simulink library "ADCS_lib"  (R2019a)
settings: Solver=VariableStepAuto  StartTime=0.0  StopTime=10.0  RelTol=1e-3
undefined symbols (not defined in the file): D_distri, G_g, G_s, G_t, Gs, I_rw, I_vscmg, I_w, J_w, K, Kc, Ki, Kp, Kv, m, OMEGA_0, P, quat_0, smiData, X, Y, Z
libraries: sm_lib x31, aerolibutil x15, nesl_utility x13, sharedtransform x4, $bdroot x2
(part 1 of 3)
settings Model: Creator=steven  LastModifiedBy=zhang
settings DataIOCC: ReturnWorkspaceOutputs=off
settings DebuggingCC: ArithmeticOperatorsInVariantConditions=warning
settings SFSimCC: SimUseLocalCustomCode=off
settings RTWCC: RTWUseLocalCustomCode=off

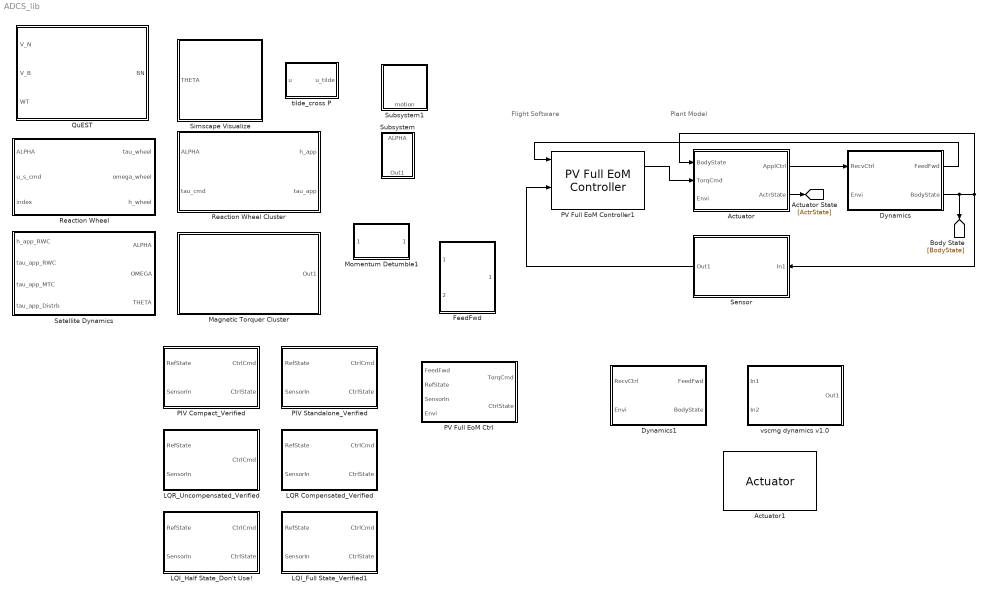
== system ADCS_lib ==
  note: Flight Software
  note: Plant Model
  Actuator : Subsystem
  Actuator1 : $bdroot/Actuator  SystemSampleTime=-1
  Dynamics : Subsystem
  Dynamics1 : Subsystem  AncestorBlock=ADCS_lib/Dynamics
  FeedFwd : Subsystem
  LQI_Full State_Verified1 : Subsystem  AncestorBlock=ADCS_lib/Full EoM Controller
      mask help:
      | Gains
      |
      | 1U
      | Kc = [eye(3).*[2.5;2.5;2.5]  eye(3).*[5;5;5]];
      | Ki  = [eye(3).*[1.2 1.2 1.2]  eye(3).*[3;3;3]];
      | Set large Ki velocity gain to surpress oscillation, x & z axis gains have the most effect
      |
      | 3U
  LQI_Half State_Don't Use! : Subsystem  AncestorBlock=ADCS_lib/Full EoM Controller
  LQR Compensated_Verified : Subsystem  AncestorBlock=ADCS_lib/PIV
  LQR_Uncompensated_Verified : Subsystem  AncestorBlock=ADCS_lib/LQR
  Magnetic Torquer Cluster : Subsystem
      mask Display: image('magnetic torquer cluster.png');
  Momentum Detumble1 : Subsystem
  PIV Compact_Verified : Subsystem  AncestorBlock=ADCS_lib/Full EoM Controller
  PIV Standalone_Verified : Subsystem  AncestorBlock=ADCS_lib/Full EoM Controller
  PV Full EoM Controller1 : $bdroot/PV Full EoM Controller  SystemSampleTime=-1  SSRTWFcnClass=[]
  PV Full EoM Ctrl : Subsystem  AncestorBlock=ADCS_lib/Full EoM Controller
  QuEST : MATLAB Function  TreatAsAtomicUnit=on  mask(QUEST Attitude Estimation){}
      mask help:
      | Estimate spacecraft attitude using QUEST algorithm
      |
      | Input: sensor measurement in inertia frame V_N
      | V_N = [x1 x2 x3 x4 x5 ... ;
      |              y1 y2 y3 y4 y5 ... ;
      |              z1 z2  z3 z4 z5 ...  ]
      |
      |             sensor measurement in body frame V_B
      | V_B = [x1 x2 x3 x4 x5 ... ;
      |             y1 y2 y3 y4 y5 ... ;
      |             z1 z2  z3 z4 z5 ...  ]
      |
      |             sensor weight wt
      | wt = [wt1 wt2 wt3 wt4 wt5 ...]
      |
      | Output: attitude [BN] in quaternion
      mask init:
      | clear all;
      | clc;
  Reaction Wheel : MATLAB Function  TreatAsAtomicUnit=on  mask(Single Reaction Wheel){}
      mask help:
      | INPUT
      | ALPHA ==> spacecraft angular acceleration (vector)
      | u_s ==> motor torque command magnitude for individual wheel in g_s direction (scalar)
      | index ==> select which wheel (1-4) (scalar)
      |
      | OUTPUT
      | tau_wheel ==> individual applied torque magnitude to spacecraft body in g_s direction (scalar)
      | omega_wheel ==> individual wheel angular velocity magnitude in g_s direction (scalar)
  Reaction Wheel Cluster : Subsystem  mask(Reaction Wheel Cluster){}
      mask Display: image('reaction wheel cluster.png');
  Satellite Dynamics : Subsystem
      mask Display: image('3u cubesat.png');
  Sensor : Subsystem
  Simscape Visualize : Subsystem
      mask Display: image('camera.png');
  Subsystem : Subsystem
  Subsystem1 : Subsystem
      mask Display: image('camera.png');
  tilde_cross P : MATLAB Function  TreatAsAtomicUnit=on
  vscmg dynamics v1.0 : Subsystem
  wires:
  ? -> PV Full EoM Controller1/2
  ? -> PV Full EoM Controller1/4, Actuator/3(Envi), Dynamics/2(Envi)
  PV Full EoM Controller1/1 -> Actuator/2(TorqCmd)
  Sensor/1(Out1) -> PV Full EoM Controller1/3
  Actuator/1(ApplCtrl) -> Dynamics/1(RecvCtrl)
  Dynamics/1(FeedFwd) -> PV Full EoM Controller1/1
  Dynamics/2(BodyState) -> Sensor/1(In1), Actuator/1(BodyState), [BodyState]
  Actuator/2(ActrState) -> [ActrState]

== system ADCS_lib/Actuator ==
  In Bus Element3 : Inport  PortName=BodyState  Element=b_a_b/n
  In Bus Element2 : Inport  PortName=BodyState  Element=b_w_b/n
  In Bus Element : Inport  Port=2  PortName=TorqCmd  Element=b_t_cmd_rwc
  In Bus Element1 : Inport  Port=2  PortName=TorqCmd  Element=b_t_cmd_mtc
  In Bus Element4 : Inport  Port=3  PortName=Envi  Element=b_t_dstb
  Magnetic Torquer Cluster : Subsystem
  Reaction Wheel Cluster : Subsystem
  Out Bus Element : Outport  PortName=ApplCtrl  Element=h_s
  Out Bus Element1 : Outport  PortName=ApplCtrl  Element=u_s
  Out Bus Element2 : Outport  PortName=ApplCtrl  Element=mtc
  Out Bus Element3 : Outport  Port=2  PortName=ActrState  Element=w_rw
  Out Bus Element4 : Outport  Port=2  PortName=ActrState  Element=t_mtc
  wires:
  In Bus Element/1 -> Reaction Wheel Cluster/3(b_t_cmd_rwc)
  In Bus Element1/1 -> Out Bus Element4/1, Magnetic Torquer Cluster/1(b_t_cmd_mtc)
  In Bus Element2/1 -> Reaction Wheel Cluster/1(b_w_b/n)
  In Bus Element3/1 -> Reaction Wheel Cluster/2(b_a_b/n)
  Reaction Wheel Cluster/1(h_s) -> Out Bus Element/1
  Reaction Wheel Cluster/2(u_s) -> Out Bus Element1/1
  Magnetic Torquer Cluster/1(Out1) -> Out Bus Element2/1
  In Bus Element4/1 -> Magnetic Torquer Cluster/2(Envi)
  Reaction Wheel Cluster/3(omega_w) -> Out Bus Element3/1

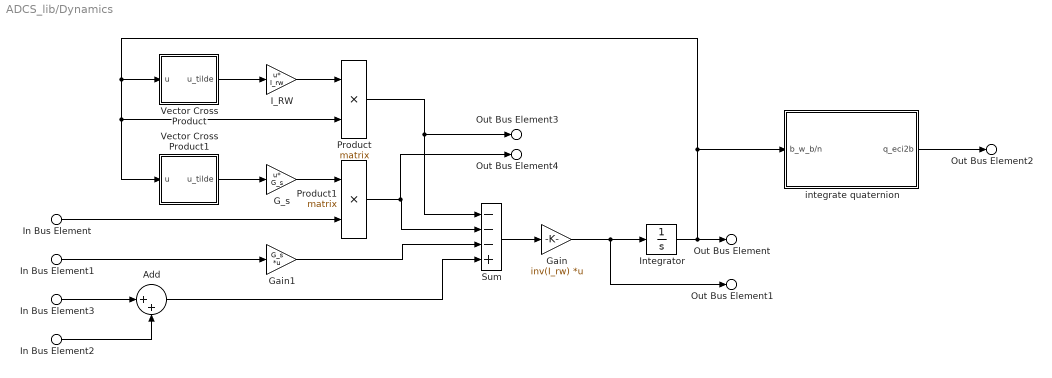
== system ADCS_lib/Dynamics ==
  In Bus Element1 : Inport  PortName=RecvCtrl  Element=u_s
  In Bus Element : Inport  PortName=RecvCtrl  Element=h_s
  In Bus Element3 : Inport  PortName=RecvCtrl  Element=mtc
  In Bus Element2 : Inport  Port=2  PortName=Envi  Element=b_t_dstb
  Add : Sum  Inputs=|++
  G_s : Gain  Gain=G_s  Multiplication=Matrix(u*K)
  Gain : Gain  Gain=inv(I_rw)  Multiplication=Matrix(K*u)
  Gain1 : Gain  Gain=G_s  Multiplication=Matrix(K*u)
  I_RW : Gain  Gain=I_rw  Multiplication=Matrix(u*K)
  Integrator : Integrator  InitialCondition=OMEGA_0
  Product : Product  Multiplication=Matrix(*)
  Product1 : Product  Multiplication=Matrix(*)
  Sum : Sum  Inputs=---+
  Vector Cross Product : MATLAB Function  TreatAsAtomicUnit=on
  Vector Cross Product1 : MATLAB Function  TreatAsAtomicUnit=on
  integrate quaternion : Subsystem
  Out Bus Element3 : Outport  PortName=FeedFwd  Element=1
  Out Bus Element4 : Outport  PortName=FeedFwd  Element=2
  Out Bus Element : Outport  Port=2  PortName=BodyState  Element=b_w_b/n
  Out Bus Element1 : Outport  Port=2  PortName=BodyState  Element=b_a_b/n
  Out Bus Element2 : Outport  Port=2  PortName=BodyState  Element=q_eci2b
  wires:
  In Bus Element2/1 -> Add/2
  Add/1 -> Sum/4
  In Bus Element3/1 -> Add/1
  Gain1/1 -> Sum/3
  In Bus Element1/1 -> Gain1/1
  Product1/1 -> Out Bus Element4/1, Sum/2
  In Bus Element/1 -> Product1/2
  G_s/1 -> Product1/1
  Vector Cross Product1/1(u_tilde) -> G_s/1
  Product/1 -> Out Bus Element3/1, Sum/1
  I_RW/1 -> Product/1
  Vector Cross Product/1(u_tilde) -> I_RW/1
  Integrator/1 -> Out Bus Element/1, integrate quaternion/1(b_w_b/n), Product/2, Vector Cross Product1/1(u), Vector Cross Product/1(u)
  Gain/1 -> Out Bus Element1/1, Integrator/1
  Sum/1 -> Gain/1
  integrate quaternion/1(q_eci2b) -> Out Bus Element2/1

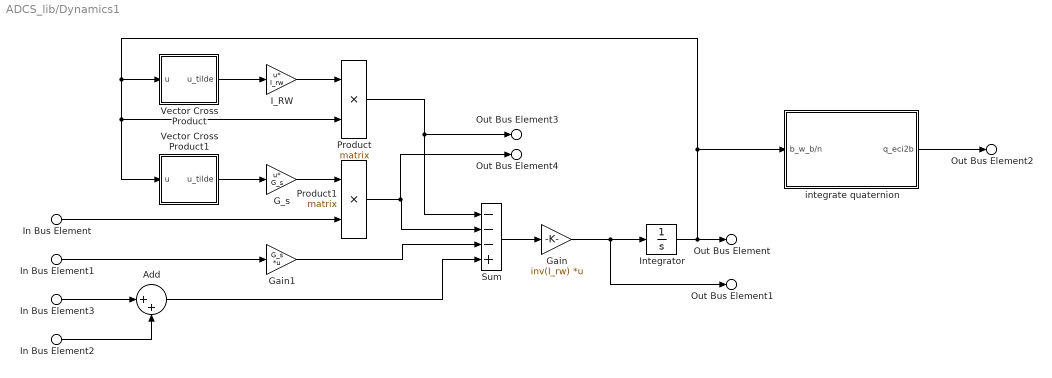
== system ADCS_lib/Dynamics1 ==
  In Bus Element1 : Inport  PortName=RecvCtrl  Element=u_s
  In Bus Element : Inport  PortName=RecvCtrl  Element=h_s
  In Bus Element3 : Inport  PortName=RecvCtrl  Element=mtc
  In Bus Element2 : Inport  Port=2  PortName=Envi  Element=b_t_dstb
  Add : Sum  Inputs=|++
  G_s : Gain  Gain=G_s  Multiplication=Matrix(u*K)
  Gain : Gain  Gain=inv(I_rw)  Multiplication=Matrix(K*u)
  Gain1 : Gain  Gain=G_s  Multiplication=Matrix(K*u)
  I_RW : Gain  Gain=I_rw  Multiplication=Matrix(u*K)
  Integrator : Integrator  InitialCondition=OMEGA_0
  Product : Product  Multiplication=Matrix(*)
  Product1 : Product  Multiplication=Matrix(*)
  Sum : Sum  Inputs=---+
  Vector Cross Product : MATLAB Function  TreatAsAtomicUnit=on
  Vector Cross Product1 : MATLAB Function  TreatAsAtomicUnit=on
  integrate quaternion : Subsystem
  Out Bus Element3 : Outport  PortName=FeedFwd  Element=1
  Out Bus Element4 : Outport  PortName=FeedFwd  Element=2
  Out Bus Element : Outport  Port=2  PortName=BodyState  Element=b_w_b/n
  Out Bus Element1 : Outport  Port=2  PortName=BodyState  Element=b_a_b/n
  Out Bus Element2 : Outport  Port=2  PortName=BodyState  Element=q_eci2b
  wires:
  integrate quaternion/1(q_eci2b) -> Out Bus Element2/1
  Sum/1 -> Gain/1
  Gain/1 -> Integrator/1, Out Bus Element1/1
  Integrator/1 -> Vector Cross Product/1(u), Vector Cross Product1/1(u), Product/2, integrate quaternion/1(b_w_b/n), Out Bus Element/1
  Vector Cross Product/1(u_tilde) -> I_RW/1
  I_RW/1 -> Product/1
  Product/1 -> Sum/1, Out Bus Element3/1
  Vector Cross Product1/1(u_tilde) -> G_s/1
  G_s/1 -> Product1/1
  In Bus Element/1 -> Product1/2
  Product1/1 -> Sum/2, Out Bus Element4/1
  In Bus Element1/1 -> Gain1/1
  Gain1/1 -> Sum/3
  In Bus Element3/1 -> Add/1
  Add/1 -> Sum/4
  In Bus Element2/1 -> Add/2

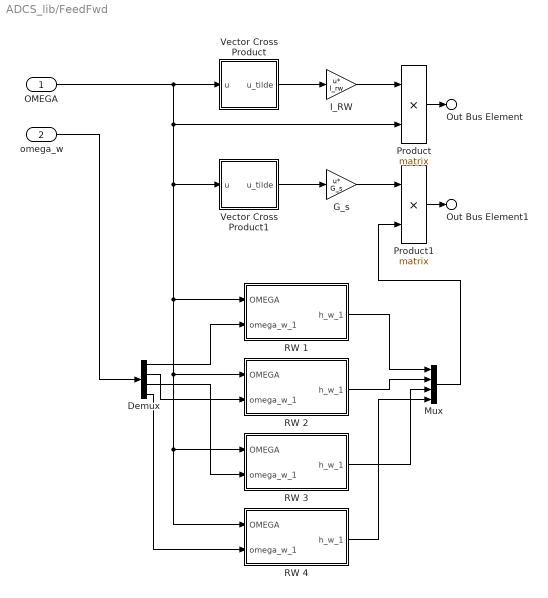
== system ADCS_lib/FeedFwd ==
  OMEGA : Inport
  omega_w : Inport  Port=2
  Demux : Demux
  G_s : Gain  Gain=G_s  Multiplication=Matrix(u*K)
  I_RW : Gain  Gain=I_rw  Multiplication=Matrix(u*K)
  Mux : Mux
  Product : Product  Multiplication=Matrix(*)
  Product1 : Product  Multiplication=Matrix(*)
  RW 1 : Subsystem
  RW 2 : Subsystem
  RW 3 : Subsystem
  RW 4 : Subsystem
  Vector Cross Product : MATLAB Function  TreatAsAtomicUnit=on
  Vector Cross Product1 : MATLAB Function  TreatAsAtomicUnit=on
  Out Bus Element : Outport  PortName=FeedFwd  Element=1
  Out Bus Element1 : Outport  PortName=FeedFwd  Element=2
  wires:
  Demux/2 -> RW 2/2(omega_w_1)
  RW 2/1(h_w_1) -> Mux/2
  Demux/4 -> RW 4/2(omega_w_1)
  OMEGA/1 -> Product/2, RW 4/1(OMEGA), RW 3/1(OMEGA), RW 2/1(OMEGA), RW 1/1(OMEGA), Vector Cross Product1/1(u), Vector Cross Product/1(u)
  Mux/1 -> Product1/2
  RW 4/1(h_w_1) -> Mux/4
  Demux/1 -> RW 1/2(omega_w_1)
  RW 1/1(h_w_1) -> Mux/1
  RW 3/1(h_w_1) -> Mux/3
  Demux/3 -> RW 3/2(omega_w_1)
  Vector Cross Product/1(u_tilde) -> I_RW/1
  Product/1 -> Out Bus Element/1
  I_RW/1 -> Product/1
  G_s/1 -> Product1/1
  Vector Cross Product1/1(u_tilde) -> G_s/1
  omega_w/1 -> Demux/1
  Product1/1 -> Out Bus Element1/1

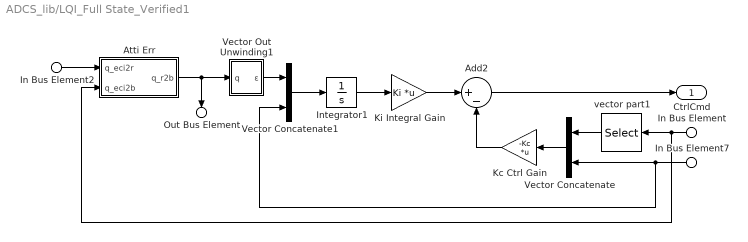
== system ADCS_lib/LQI_Full State_Verified1 ==
  In Bus Element2 : Inport  PortName=RefState  Element=q_eci2r
  In Bus Element : Inport  Port=2  PortName=SensorIn  Element=q_eci2b
  In Bus Element7 : Inport  Port=2  PortName=SensorIn  Element=b_w_b/n
  Add2 : Sum  Inputs=|+-
  Atti Err : Subsystem  AncestorBlock=ADCS_lib/PIV/Atti Err
  Integrator1 : Integrator
  Kc Ctrl Gain : Gain  Gain=-Kc  Multiplication=Matrix(K*u)
  Ki Integral Gain : Gain  Gain=Ki  Multiplication=Matrix(K*u)
  Vector Concatenate : Concatenate
  Vector Concatenate1 : Concatenate
  Vector Out Unwinding1 : Subsystem
  vector part1 : Selector  InputPortWidth=4  IndexOptions=Index vector (dialog)  Indices=[2 3 4]  OutputSizes=1
  CtrlCmd : Outport
  Out Bus Element : Outport  Port=2  PortName=CtrlState  Element=q_r2b
  wires:
  Vector Concatenate1/1 -> Integrator1/1
  Vector Out Unwinding1/1(ε) -> Vector Concatenate1/1
  In Bus Element7/1 -> Vector Concatenate1/2, Vector Concatenate/2
  Vector Concatenate/1 -> Kc Ctrl Gain/1
  vector part1/1 -> Vector Concatenate/1
  Integrator1/1 -> Ki Integral Gain/1
  Add2/1 -> CtrlCmd/1
  Kc Ctrl Gain/1 -> Add2/2
  In Bus Element2/1 -> Atti Err/1(q_eci2r)
  In Bus Element/1 -> Atti Err/2(q_eci2b), vector part1/1
  Atti Err/1(q_r2b) -> Vector Out Unwinding1/1(q), Out Bus Element/1
  Ki Integral Gain/1 -> Add2/1

== system ADCS_lib/LQI_Half State_Don't Use! ==
  In Bus Element2 : Inport  PortName=RefState  Element=q_eci2r
  In Bus Element : Inport  Port=2  PortName=SensorIn  Element=q_eci2b
  In Bus Element7 : Inport  Port=2  PortName=SensorIn  Element=b_w_b/n
  Add2 : Sum  Inputs=|+-
  Atti Err1 : Subsystem
  Integrator1 : Integrator
  Kc Ctrl Gain : Gain  Gain=-Kc  Multiplication=Matrix(K*u)
  Ki Integral Gain : Gain  Gain=Ki  Multiplication=Matrix(K*u)
  Vector Concatenate : Concatenate
  Vector Out Unwinding2 : Subsystem
  vector part : Selector  InputPortWidth=4  IndexOptions=Index vector (dialog)  Indices=[2 3 4]  OutputSizes=1
  CtrlCmd : Outport
  Out Bus Element : Outport  Port=2  PortName=CtrlState  Element=q_r2b
  wires:
  In Bus Element7/1 -> Vector Concatenate/2
  Vector Concatenate/1 -> Kc Ctrl Gain/1
  vector part/1 -> Vector Concatenate/1
  Integrator1/1 -> Ki Integral Gain/1
  Add2/1 -> CtrlCmd/1
  Kc Ctrl Gain/1 -> Add2/2
  In Bus Element2/1 -> Atti Err1/1(q_eci2r)
  In Bus Element/1 -> vector part/1, Atti Err1/2(q_eci2b)
  Atti Err1/1(q_r2b) -> Vector Out Unwinding2/1(q), Out Bus Element/1
  Vector Out Unwinding2/1(ε) -> Integrator1/1
  Ki Integral Gain/1 -> Add2/1

== system ADCS_lib/LQR Compensated_Verified ==
  In Bus Element1 : Inport  PortName=RefState  Element=q_eci2r
  In Bus Element4 : Inport  PortName=RefState  Element=r_w_r/n
  In Bus Element : Inport  Port=2  PortName=SensorIn  Element=q_eci2b
  In Bus Element7 : Inport  Port=2  PortName=SensorIn  Element=b_w_b/n
  Add1 : Sum  Inputs=|-+
  Atti Err : Subsystem
  Kc Ctrl Gain Mtx : Gain  Gain=Kc  Multiplication=Matrix(K*u)
  Terminator : Terminator
  Vector Concatenate : Concatenate
  Vector Out Unwinding : Subsystem
  r2b : Subsystem
  CtrlCmd : Outport
  Out Bus Element : Outport  Port=2  PortName=CtrlState  Element=q_r2b
  Out Bus Element1 : Outport  Port=2  PortName=CtrlState  Element=b_w_b/r
  wires:
  In Bus Element4/1 -> r2b/2(r_w_r/n)
  Atti Err/2(DCM) -> r2b/1("[BR]")
  Atti Err/1(q_r2b) -> Vector Out Unwinding/1(q), Out Bus Element/1  "q_r2b"
  In Bus Element1/1 -> Atti Err/1(q_eci2r)
  In Bus Element/1 -> Atti Err/2(q_eci2b)
  In Bus Element7/1 -> Add1/2
  r2b/1(b_w_r/n) -> Add1/1
  Add1/1 -> Vector Concatenate/2, Out Bus Element1/1  "b_w_b/r"
  r2b/2(b_a_r/n) -> Terminator/1
  Vector Concatenate/1 -> Kc Ctrl Gain Mtx/1
  Kc Ctrl Gain Mtx/1 -> CtrlCmd/1
  Vector Out Unwinding/1(ε) -> Vector Concatenate/1

== system ADCS_lib/LQR_Uncompensated_Verified ==
  In Bus Element2 : Inport  PortName=RefState  Element=q_eci2r
  In Bus Element : Inport  Port=2  PortName=SensorIn  Element=q_eci2b
  In Bus Element7 : Inport  Port=2  PortName=SensorIn  Element=b_w_b/n
  Add2 : Sum  Inputs=|+-
  Kc Ctrl Gain : Gain  Gain=-Kc  Multiplication=Matrix(K*u)
  Vector Concatenate : Concatenate
  vector part : Selector  InputPortWidth=4  IndexOptions=Index vector (dialog)  Indices=[2 3 4]  OutputSizes=1
  vector part1 : Selector  InputPortWidth=4  IndexOptions=Index vector (dialog)  Indices=[2 3 4]  OutputSizes=1
  CtrlCmd : Outport
  wires:
  In Bus Element7/1 -> Vector Concatenate/2
  Vector Concatenate/1 -> Kc Ctrl Gain/1
  Add2/1 -> CtrlCmd/1
  Kc Ctrl Gain/1 -> Add2/2
  In Bus Element2/1 -> vector part1/1
  vector part1/1 -> Add2/1
  In Bus Element/1 -> vector part/1
  vector part/1 -> Vector Concatenate/1

== system ADCS_lib/Magnetic Torquer Cluster ==
  Constant : Constant  Value=[0;0;0]
  Out1 : Outport
  wires:
  Constant/1 -> Out1/1

== system ADCS_lib/Momentum Detumble1 ==
  OMEGA : Inport
  Detumble Gain : Gain  Gain=-[1 0 0;0 1 0;0 0 1]  Multiplication=Matrix(K*u)
  I_rw : Gain  Gain=I_rw  Multiplication=Matrix(K*u)
  tau_ext : Outport
  wires:
  Detumble Gain/1 -> tau_ext/1
  OMEGA/1 -> I_rw/1
  I_rw/1 -> Detumble Gain/1

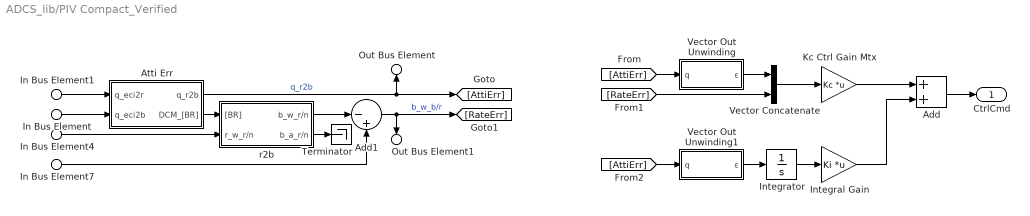
== system ADCS_lib/PIV Compact_Verified ==
  In Bus Element1 : Inport  PortName=RefState  Element=q_eci2r
  In Bus Element4 : Inport  PortName=RefState  Element=r_w_r/n
  In Bus Element : Inport  Port=2  PortName=SensorIn  Element=q_eci2b
  In Bus Element7 : Inport  Port=2  PortName=SensorIn  Element=b_w_b/n
  Add : Sum
  Add1 : Sum  Inputs=|-+
  Atti Err : Subsystem
  Integral Gain : Gain  Gain=Ki  Multiplication=Matrix(K*u)
  Integrator : Integrator
  Kc Ctrl Gain Mtx : Gain  Gain=Kc  Multiplication=Matrix(K*u)
  Terminator : Terminator
  Vector Concatenate : Concatenate
  Vector Out Unwinding : Subsystem
  Vector Out Unwinding1 : Subsystem
  r2b : Subsystem
  CtrlCmd : Outport
  Out Bus Element : Outport  Port=2  PortName=CtrlState  Element=q_r2b
  Out Bus Element1 : Outport  Port=2  PortName=CtrlState  Element=b_w_b/r
  wires:
  Integrator/1 -> Integral Gain/1
  In Bus Element4/1 -> r2b/2(r_w_r/n)
  Atti Err/2(DCM_[BR]) -> r2b/1("[BR]")
  Atti Err/1(q_r2b) -> Out Bus Element/1, [AttiErr]  "q_r2b"
  In Bus Element1/1 -> Atti Err/1(q_eci2r)
  In Bus Element/1 -> Atti Err/2(q_eci2b)
  In Bus Element7/1 -> Add1/2
  r2b/1(b_w_r/n) -> Add1/1
  Add1/1 -> Out Bus Element1/1, [RateErr]  "b_w_b/r"
  r2b/2(b_a_r/n) -> Terminator/1
  [RateErr] -> Vector Concatenate/2
  Vector Concatenate/1 -> Kc Ctrl Gain Mtx/1
  Kc Ctrl Gain Mtx/1 -> Add/1
  Add/1 -> CtrlCmd/1
  Vector Out Unwinding1/1(ε) -> Integrator/1
  Integral Gain/1 -> Add/2
  [AttiErr] -> Vector Out Unwinding/1(q)
  Vector Out Unwinding/1(ε) -> Vector Concatenate/1
  [AttiErr] -> Vector Out Unwinding1/1(q)

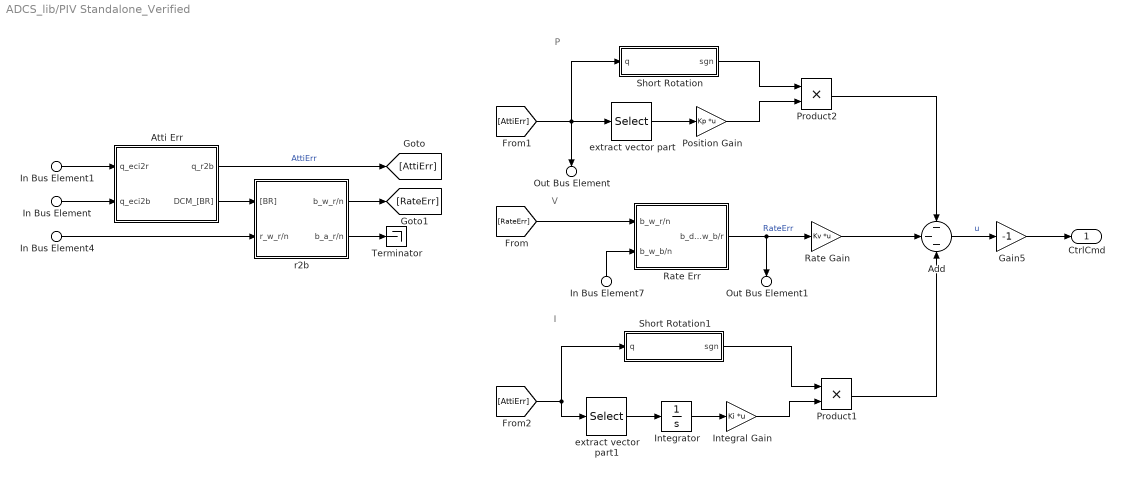
== system ADCS_lib/PIV Standalone_Verified ==
  note: P
  note: V
  note: I
  In Bus Element1 : Inport  PortName=RefState  Element=q_eci2r
  In Bus Element4 : Inport  PortName=RefState  Element=r_w_r/n
  In Bus Element : Inport  Port=2  PortName=SensorIn  Element=q_eci2b
  In Bus Element7 : Inport  Port=2  PortName=SensorIn  Element=b_w_b/n
  Add : Sum  Inputs=---
  Atti Err : Subsystem
  Gain5 : Gain  Gain=-1
  Integral Gain : Gain  Gain=Ki  Multiplication=Matrix(K*u)
  Integrator : Integrator
  Position Gain : Gain  Gain=Kp  Multiplication=Matrix(K*u)
  Product1 : Product
  Product2 : Product
  Rate Err : Subsystem
  Rate Gain : Gain  Gain=Kv  Multiplication=Matrix(K*u)
  Short Rotation : Subsystem
  Short Rotation1 : Subsystem
  Terminator : Terminator
  extract vector part : Selector  InputPortWidth=4  IndexOptions=Index vector (dialog)  Indices=[2 3 4]  OutputSizes=1
  extract vector part1 : Selector  InputPortWidth=4  IndexOptions=Index vector (dialog)  Indices=[2 3 4]  OutputSizes=1
  r2b : Subsystem
  CtrlCmd : Outport
  Out Bus Element : Outport  Port=2  PortName=CtrlState  Element=q_r2b
  Out Bus Element1 : Outport  Port=2  PortName=CtrlState  Element=deltaw_b/r
  wires:
  extract vector part1/1 -> Integrator/1
  Integrator/1 -> Integral Gain/1
  Integral Gain/1 -> Product1/2
  Short Rotation1/1(sgn) -> Product1/1
  Product1/1 -> Add/3
  [AttiErr] -> Short Rotation1/1(q), extract vector part1/1
  r2b/1(b_w_r/n) -> [RateErr]
  [RateErr] -> Rate Err/1(b_w_r/n)
  [AttiErr] -> Out Bus Element/1, Short Rotation/1(q), extract vector part/1
  Short Rotation/1(sgn) -> Product2/1
  Product2/1 -> Add/1
  Position Gain/1 -> Product2/2
  Rate Gain/1 -> Add/2
  Rate Err/1(b_deltaw_b/r) -> Out Bus Element1/1, Rate Gain/1  "RateErr"
  In Bus Element7/1 -> Rate Err/2(b_w_b/n)
  extract vector part/1 -> Position Gain/1
  In Bus Element4/1 -> r2b/2(r_w_r/n)
  Atti Err/2(DCM_[BR]) -> r2b/1("[BR]")
  Atti Err/1(q_r2b) -> [AttiErr]  "AttiErr"
  In Bus Element1/1 -> Atti Err/1(q_eci2r)
  In Bus Element/1 -> Atti Err/2(q_eci2b)
  Gain5/1 -> CtrlCmd/1
  Add/1 -> Gain5/1  "u"
  r2b/2(b_a_r/n) -> Terminator/1

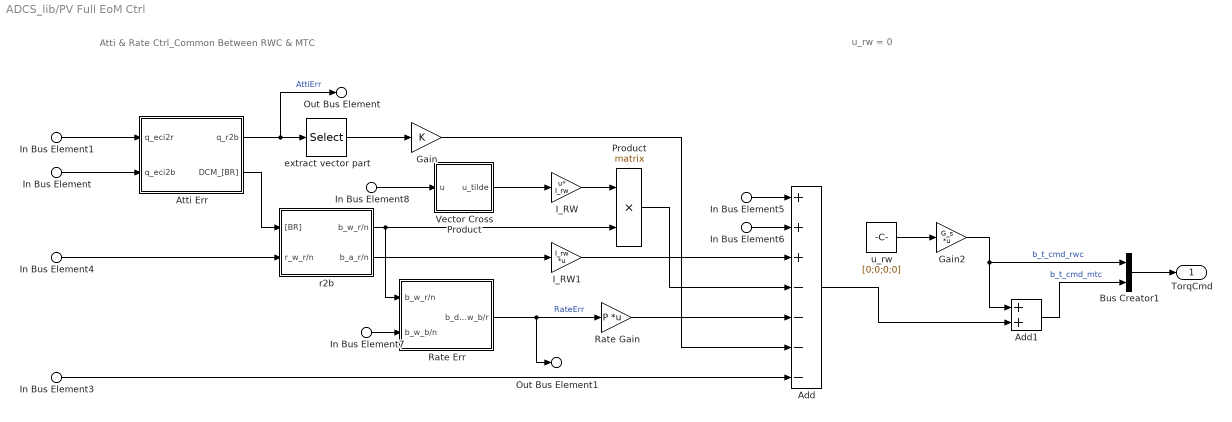
== system ADCS_lib/PV Full EoM Ctrl ==
  note: u_rw = 0
  note: Atti & Rate Ctrl_Common Between RWC & MTC
  In Bus Element5 : Inport  PortName=FeedFwd  Element=1
  In Bus Element6 : Inport  PortName=FeedFwd  Element=2
  In Bus Element1 : Inport  Port=2  PortName=RefState  Element=q_eci2r
  In Bus Element4 : Inport  Port=2  PortName=RefState  Element=r_w_r/n
  In Bus Element : Inport  Port=3  PortName=SensorIn  Element=q_eci2b
  In Bus Element7 : Inport  Port=3  PortName=SensorIn  Element=b_w_b/n
  In Bus Element8 : Inport  Port=3  PortName=SensorIn  Element=b_w_b/n
  In Bus Element3 : Inport  Port=4  PortName=Envi  Element=b_t_dstb
  Add : Sum  Inputs=+++----
  Add1 : Sum
  Atti Err : Subsystem
  Bus Creator1 : BusCreator  Inputs=2
  Gain : Gain  Gain=K
  Gain2 : Gain  Gain=G_s  Multiplication=Matrix(K*u)
  I_RW : Gain  Gain=I_rw  Multiplication=Matrix(u*K)
  I_RW1 : Gain  Gain=I_rw  Multiplication=Matrix(K*u)
  Product : Product  Multiplication=Matrix(*)
  Rate Err : Subsystem
  Rate Gain : Gain  Gain=P  Multiplication=Matrix(K*u)
  Vector Cross Product : MATLAB Function  TreatAsAtomicUnit=on
  extract vector part : Selector  InputPortWidth=4  IndexOptions=Index vector (dialog)  Indices=[2 3 4]  OutputSizes=1
  r2b : Subsystem
  u_rw : Constant  Value=[0;0;0;0]
  TorqCmd : Outport
  Out Bus Element : Outport  Port=2  PortName=CtrlState  Element=q_r2b
  Out Bus Element1 : Outport  Port=2  PortName=CtrlState  Element=deltaw_b/r
  wires:
  In Bus Element6/1 -> Add/2
  In Bus Element5/1 -> Add/1
  Gain2/1 -> Bus Creator1/1, Add1/1  "b_t_cmd_rwc"
  Add/1 -> Add1/2
  u_rw/1 -> Gain2/1
  Add1/1 -> Bus Creator1/2  "b_t_cmd_mtc"
  Bus Creator1/1 -> TorqCmd/1
  I_RW1/1 -> Add/3
  r2b/2(b_a_r/n) -> I_RW1/1
  Product/1 -> Add/4
  Vector Cross Product/1(u_tilde) -> I_RW/1
  In Bus Element8/1 -> Vector Cross Product/1(u)
  I_RW/1 -> Product/1
  r2b/1(b_w_r/n) -> Product/2, Rate Err/1(b_w_r/n)
  Rate Gain/1 -> Add/5
  Rate Err/1(b_deltaw_b/r) -> Out Bus Element1/1, Rate Gain/1  "RateErr"
  In Bus Element7/1 -> Rate Err/2(b_w_b/n)
  Gain/1 -> Add/6
  extract vector part/1 -> Gain/1
  In Bus Element4/1 -> r2b/2(r_w_r/n)
  Atti Err/2(DCM_[BR]) -> r2b/1("[BR]")
  In Bus Element1/1 -> Atti Err/1(q_eci2r)
  In Bus Element/1 -> Atti Err/2(q_eci2b)
  In Bus Element3/1 -> Add/7
  Atti Err/1(q_r2b) -> Out Bus Element/1, extract vector part/1  "AttiErr"

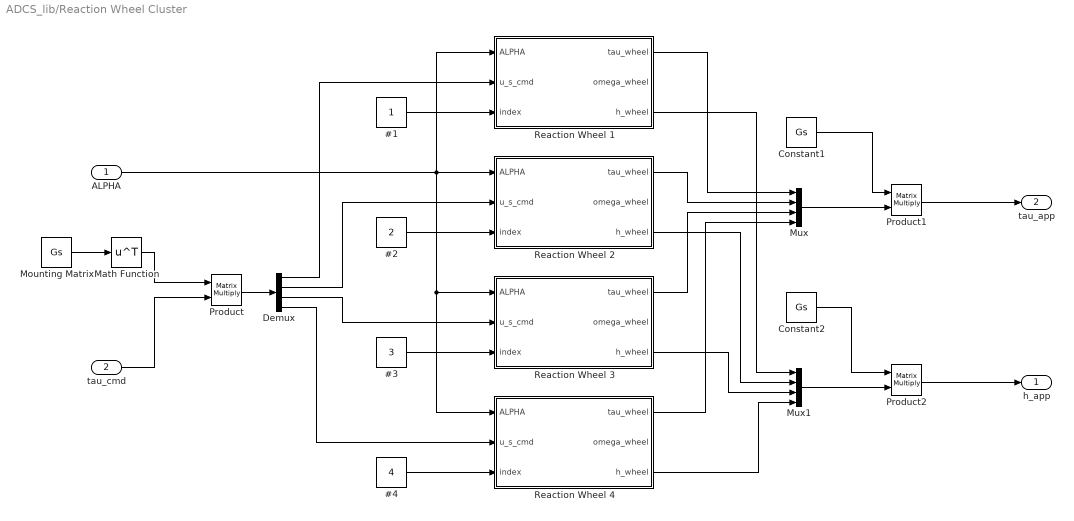
== system ADCS_lib/Reaction Wheel Cluster ==
  ALPHA : Inport
  tau_cmd : Inport  Port=2
  #1 : Constant
  #2 : Constant  Value=2
  #3 : Constant  Value=3
  #4 : Constant  Value=4
  Constant1 : Constant  Value=Gs
  Constant2 : Constant  Value=Gs
  Demux : Demux
  Math Function : Math  Operator=transpose  SaturateOnIntegerOverflow=on
  Mounting Matrix : Constant  Value=Gs
  Mux : Mux
  Mux1 : Mux
  Product : Product  Multiplication=Matrix(*)
  Product1 : Product  Multiplication=Matrix(*)
  Product2 : Product  Multiplication=Matrix(*)
  Reaction Wheel 1 : MATLAB Function  TreatAsAtomicUnit=on  mask(Single Reaction Wheel){Gs=Gs, J_w=J_w}
      mask prompts: Gs "mounting matrix in spin direction"; J_w "wheel inertia matrix"
      mask help:
      | INPUT
      | ALPHA ==> spacecraft angular acceleration (vector)
      | u_s ==> motor torque command magnitude for individual wheel in g_s direction (scalar)
      | index ==> select which wheel (1-4) (scalar)
      |
      | OUTPUT
      | tau_wheel ==> individual applied torque magnitude to spacecraft body in g_s direction (scalar)
      | omega_wheel ==> individual wheel angular velocity magnitude in g_s direction (scalar)
  Reaction Wheel 2 : MATLAB Function  TreatAsAtomicUnit=on  mask(Single Reaction Wheel){}
      mask help:
      | INPUT
      | ALPHA ==> spacecraft angular acceleration (vector)
      | u_s ==> motor torque command magnitude for individual wheel in g_s direction (scalar)
      | index ==> select which wheel (1-4) (scalar)
      |
      | OUTPUT
      | tau_wheel ==> individual applied torque magnitude to spacecraft body in g_s direction (scalar)
      | omega_wheel ==> individual wheel angular velocity magnitude in g_s direction (scalar)
  Reaction Wheel 3 : MATLAB Function  TreatAsAtomicUnit=on  mask(Single Reaction Wheel){}
      mask help:
      | INPUT
      | ALPHA ==> spacecraft angular acceleration (vector)
      | u_s ==> motor torque command magnitude for individual wheel in g_s direction (scalar)
      | index ==> select which wheel (1-4) (scalar)
      |
      | OUTPUT
      | tau_wheel ==> individual applied torque magnitude to spacecraft body in g_s direction (scalar)
      | omega_wheel ==> individual wheel angular velocity magnitude in g_s direction (scalar)
  Reaction Wheel 4 : MATLAB Function  TreatAsAtomicUnit=on  mask(Single Reaction Wheel){}
      mask help:
      | INPUT
      | ALPHA ==> spacecraft angular acceleration (vector)
      | u_s ==> motor torque command magnitude for individual wheel in g_s direction (scalar)
      | index ==> select which wheel (1-4) (scalar)
      |
      | OUTPUT
      | tau_wheel ==> individual applied torque magnitude to spacecraft body in g_s direction (scalar)
      | omega_wheel ==> individual wheel angular velocity magnitude in g_s direction (scalar)
  h_app : Outport
  tau_app : Outport  Port=2
  wires:
  #1/1 -> Reaction Wheel 1/3(index)
  #2/1 -> Reaction Wheel 2/3(index)
  #3/1 -> Reaction Wheel 3/3(index)
  #4/1 -> Reaction Wheel 4/3(index)
  ALPHA/1 -> Reaction Wheel 1/1(ALPHA), Reaction Wheel 2/1(ALPHA), Reaction Wheel 4/1(ALPHA), Reaction Wheel 3/1(ALPHA)
  tau_cmd/1 -> Product/2
  Mounting Matrix/1 -> Math Function/1
  Math Function/1 -> Product/1
  Product/1 -> Demux/1
  Demux/1 -> Reaction Wheel 1/2(u_s_cmd)
  Demux/2 -> Reaction Wheel 2/2(u_s_cmd)
  Demux/4 -> Reaction Wheel 4/2(u_s_cmd)
  Demux/3 -> Reaction Wheel 3/2(u_s_cmd)
  Reaction Wheel 1/1(tau_wheel) -> Mux/1
  Reaction Wheel 2/1(tau_wheel) -> Mux/2
  Reaction Wheel 3/1(tau_wheel) -> Mux/3
  Reaction Wheel 4/1(tau_wheel) -> Mux/4
  Mux/1 -> Product1/2
  Constant1/1 -> Product1/1
  Product1/1 -> tau_app/1
  Constant2/1 -> Product2/1
  Mux1/1 -> Product2/2
  Reaction Wheel 1/3(h_wheel) -> Mux1/1
  Reaction Wheel 2/3(h_wheel) -> Mux1/2
  Reaction Wheel 3/3(h_wheel) -> Mux1/3
  Reaction Wheel 4/3(h_wheel) -> Mux1/4
  Product2/1 -> h_app/1

== system ADCS_lib/Satellite Dynamics ==
  h_app_RWC : Inport
  tau_app_RWC : Inport  Port=2
  tau_app_MTC : Inport  Port=3
  tau_app_Distrb : Inport  Port=4
  Equation of Motion : MATLAB Function  TreatAsAtomicUnit=on
  Integrator : Integrator
  Integrator1 : Integrator
  Sum : Sum  Inputs=|++
  ALPHA : Outport
  OMEGA : Outport  Port=2
  THETA : Outport  Port=3
  wires:
  Equation of Motion/1(ALPHA) -> ALPHA/1, Integrator/1
  Integrator/1 -> Integrator1/1, Equation of Motion/1(OMEGA), OMEGA/1
  Integrator1/1 -> THETA/1
  h_app_RWC/1 -> Equation of Motion/2(h_app_RWC)
  tau_app_RWC/1 -> Equation of Motion/3(tau_app_RWC)
  tau_app_MTC/1 -> Sum/1
  tau_app_Distrb/1 -> Sum/2
  Sum/1 -> Equation of Motion/4(tau_app_distrb)

== system ADCS_lib/Sensor ==
  In1 : Inport
  Out1 : Outport
  wires:
  In1/1 -> Out1/1

== system ADCS_lib/Simscape Visualize ==
  note: Initial tip off angular velocities range from -5 to 5 deg/s
  note: Deployment velocity ranges 0.5 to 2 m/s
  THETA : Inport
  CubeSat : sm_lib/Body Elements/Solid  InertiaType=Custom  Mass=m  MassUnits=kg  CenterOfMass=CoM  CenterOfMassUnits=mm  MomentsOfInertia=MoI  MomentsOfInertiaUnits=g*mm^2  ProductsOfInertia=PoI  ProductsOfInertiaUnits=g*mm^2  BasedOnType=Density  Density=1000  DensityUnits=kg/m^3  DoExposeReferenceFrame=on  SerializedFrames=<Frames><Frame><Id>Frame1</Id><Value><Name>F1</Name><Origin><Source>CenterOfMassFrame</Source><FeatureName></FeatureName></Origin><PrimaryAxis><DefinedDirection>+Z</DefinedDirection><Source>ReferenceFrame</Source><SourceDirection>+Z</SourceDirection><FeatureName></FeatureName></PrimaryAxis><SecondaryAxis><DefinedDirection>+X</DefinedDirection><Source>ReferenceFrame</Source><SourceDirection>+X</SourceDirection><FeatureName></FeatureName></SecondaryAxis></Value></Frame></Frames>  GraphicType=FromGeometry  MarkerShape=Sphere  MarkerSize=10  GraphicVisPropType=SimpleVisualProperties  GraphicDiffuseColor=[0.5 0.5 0.5]  GraphicSpecularColor=[0.5 0.5 0.5 1.0]  GraphicAmbientColor=[0.15 0.15 0.15 1.0]  GraphicEmissiveColor=[0.0 0.0 0.0 1.0]  GraphicShininess=75  GraphicOpacity=1.0  GeometryShape=FromFile  RectangleSize=[1 1]  RectangleSizeUnits=m  BrickDimensions=[1 1 1]  BrickDimensionUnits=m  CylinderRadius=1  CylinderRadiusUnits=m  CylinderLength=1  CylinderLengthUnits=m  SphereRadius=1  SphereRadiusUnits=m  EllipsoidRadii=[1 1 1]  EllipsoidRadiiUnits=m  ExtrusionCrossSection=[1 1; -1 1; -1 -1; 1 -1]  ExtrusionCrossSectionUnits=m  ExtrusionLength=1  ExtrusionLengthUnits=m  PolygonNumSides=3  PolygonOuterRadius=1  PolygonOuterRadiusUnits=m  ExtGeomFileType=STEP  ExtGeomFileName=.\Cubesat_Model.STEP  ExtGeomFileUnits=m  RevolutionCrossSection=[1 1; 1 -1; 2 -1; 2 1]  RevolutionCrossSectionUnits=m  RevolutionExtent=Full  RevolutionAngle=180  RevolutionAngleUnits=deg
  Demux : Demux  Outputs=3
  Gain : Gain  Commented=on  Gain=57.2958
  Gimbal Joint : sm_lib/Joints/Gimbal Joint  SenseConstraintForce=off  SenseConstraintForceX=off  SenseConstraintForceY=off  SenseConstraintForceZ=off  SenseConstraintTorque=off  SenseConstraintTorqueX=off  SenseConstraintTorqueY=off  SenseConstraintTorqueZ=off  SenseTotalForce=off  SenseTotalForceX=off  SenseTotalForceY=off  SenseTotalForceZ=off  SenseTotalTorque=off  SenseTotalTorqueX=off  SenseTotalTorqueY=off  SenseTotalTorqueZ=off  CompositeWrenchDir=FollowerOnBase  CompositeWrenchFrame=BaseFrame  RxEquilibriumPosition=0  RxEquilibriumPositionUnits=deg  RxSpringStiffness=0  RxSpringStiffnessUnits=N*m/deg  RxDampingCoefficient=0  RxDampingCoefficientUnits=N*m/(deg/s)  RxTorqueActuationMode=NoTorque  RxMotionActuationMode=InputMotion  RxSensePosition=off  RxSenseVelocity=off  RxSenseAcceleration=off  RxSenseTorqueForce=off  RxSenseLowerLimitTorqueForce=off  RxSenseUpperLimitTorqueForce=off  RxLowerLimitSpecify=off  RxLowerLimitBound=-90  RxLowerLimitBoundUnits=deg  RxLowerLimitStiffness=1e4  RxLowerLimitStiffnessUnits=N*m/deg  RxLowerLimitDamping=10  RxLowerLimitDampingUnits=N*m/(deg/s)  RxLowerLimitTransitionRegionWidth=0.1  RxLowerLimitTransitionRegionWidthUnits=deg  RxUpperLimitSpecify=off  RxUpperLimitBound=90  RxUpperLimitBoundUnits=deg  RxUpperLimitStiffness=1e4  RxUpperLimitStiffnessUnits=N*m/deg  RxUpperLimitDamping=10  RxUpperLimitDampingUnits=N*m/(deg/s)  RxUpperLimitTransitionRegionWidth=0.1  RxUpperLimitTransitionRegionWidthUnits=deg  RxPositionTargetSpecify=off  RxPositionTargetPriority=High  RxPositionTargetValue=0  RxPositionTargetValueUnits=deg  RxVelocityTargetSpecify=off  RxVelocityTargetPriority=High  RxVelocityTargetValue=0  RxVelocityTargetValueUnits=deg/s  RyEquilibriumPosition=0  RyEquilibriumPositionUnits=deg  RySpringStiffness=0  RySpringStiffnessUnits=N*m/deg  RyDampingCoefficient=0  RyDampingCoefficientUnits=N*m/(deg/s)  RyTorqueActuationMode=NoTorque  RyMotionActuationMode=InputMotion  RySensePosition=off  RySenseVelocity=off  RySenseAcceleration=off  RySenseTorqueForce=off  RySenseLowerLimitTorqueForce=off  RySenseUpperLimitTorqueForce=off  RyLowerLimitSpecify=off  RyLowerLimitBound=-90  RyLowerLimitBoundUnits=deg  RyLowerLimitStiffness=1e4  RyLowerLimitStiffnessUnits=N*m/deg  RyLowerLimitDamping=10  RyLowerLimitDampingUnits=N*m/(deg/s)  RyLowerLimitTransitionRegionWidth=0.1  RyLowerLimitTransitionRegionWidthUnits=deg  RyUpperLimitSpecify=off  RyUpperLimitBound=90  RyUpperLimitBoundUnits=deg  RyUpperLimitStiffness=1e4  RyUpperLimitStiffnessUnits=N*m/deg  RyUpperLimitDamping=10  RyUpperLimitDampingUnits=N*m/(deg/s)  RyUpperLimitTransitionRegionWidth=0.1  RyUpperLimitTransitionRegionWidthUnits=deg  RyPositionTargetSpecify=off  RyPositionTargetPriority=High  RyPositionTargetValue=0  RyPositionTargetValueUnits=deg  RyVelocityTargetSpecify=off  RyVelocityTargetPriority=High  RyVelocityTargetValue=0  RyVelocityTargetValueUnits=deg/s  RzEquilibriumPosition=0  RzEquilibriumPositionUnits=deg  RzSpringStiffness=0  RzSpringStiffnessUnits=N*m/deg  RzDampingCoefficient=0  RzDampingCoefficientUnits=N*m/(deg/s)  RzTorqueActuationMode=NoTorque  RzMotionActuationMode=InputMotion  RzSensePosition=off  RzSenseVelocity=off  RzSenseAcceleration=off  RzSenseTorqueForce=off  RzSenseLowerLimitTorqueForce=off  RzSenseUpperLimitTorqueForce=off  RzLowerLimitSpecify=off  RzLowerLimitBound=-90  RzLowerLimitBoundUnits=deg  RzLowerLimitStiffness=1e4  RzLowerLimitStiffnessUnits=N*m/deg  RzLowerLimitDamping=10  RzLowerLimitDampingUnits=N*m/(deg/s)  RzLowerLimitTransitionRegionWidth=0.1  RzLowerLimitTransitionRegionWidthUnits=deg  RzUpperLimitSpecify=off  RzUpperLimitBound=90  RzUpperLimitBoundUnits=deg  RzUpperLimitStiffness=1e4  RzUpperLimitStiffnessUnits=N*m/deg  RzUpperLimitDamping=10  RzUpperLimitDampingUnits=N*m/(deg/s)  RzUpperLimitTransitionRegionWidth=0.1  RzUpperLimitTransitionRegionWidthUnits=deg  RzPositionTargetSpecify=off  RzPositionTargetPriority=High  RzPositionTargetValue=0  RzPositionTargetValueUnits=deg  RzVelocityTargetSpecify=off  RzVelocityTargetPriority=High  RzVelocityTargetValue=0  RzVelocityTargetValueUnits=deg/s
      settings: SourceProductName=Simscape Multibody
  Mechanism Configuration : sm_lib/Utilities/Mechanism Configuration  UniformGravity=None  GravityVector=[0 0 -9.80665]  GravityUnits=m/s^2  LinearizationDelta=0.001
  PS-Simulink Converter : nesl_utility/PS-Simulink Converter  Commented=on  PhysicalDomain=network_engine_domain  SubClassName=ps_output  LeftPortType=input  RightPortType=output  PseudoPeriodic=off  Frequencies=[]  Unit=1  AffineConversion=off
  Simulink-PS Converter : nesl_utility/Simulink-PS Converter  PhysicalDomain=network_engine_domain  SubClassName=ps_input  LeftPortType=input  RightPortType=output  PseudoPeriodic=off  Frequencies=[]  NoiseDistribution=none  NoiseParameters=[]  Unit=1  AffineConversion=off  FilteringAndDerivatives=provide  SimscapeFilterOrder=1  InputFilterTimeConstant=0.001  UdotUserProvided=0
  Simulink-PS Converter1 : nesl_utility/Simulink-PS Converter  PhysicalDomain=network_engine_domain  SubClassName=ps_input  LeftPortType=input  RightPortType=output  PseudoPeriodic=off  Frequencies=[]  NoiseDistribution=none  NoiseParameters=[]  Unit=1  AffineConversion=off  FilteringAndDerivatives=provide  SimscapeFilterOrder=1  InputFilterTimeConstant=0.001  UdotUserProvided=0
  Simulink-PS Converter2 : nesl_utility/Simulink-PS Converter  PhysicalDomain=network_engine_domain  SubClassName=ps_input  LeftPortType=input  RightPortType=output  PseudoPeriodic=off  Frequencies=[]  NoiseDistribution=none  NoiseParameters=[]  Unit=1  AffineConversion=off  FilteringAndDerivatives=provide  SimscapeFilterOrder=1  InputFilterTimeConstant=0.001  UdotUserProvided=0
  Solver Configuration : nesl_utility/Solver Configuration  PhysicalDomain=network_engine_domain  SubClassName=solver  LeftPortType=input  RightPortType=generic  Tones=[]  Harmonics=[]  SimulateNoise=off  Profile=off  UseLocalSampling=off  EnableSwitchedLinearOptims=on  FrequencyDomain=off  UseCCode=off  RelTol=0.001  AbsTol=1e-06  MinStep=1e-09  ToWorkspace=off  RevertToSquareIcSolve=off  NumHomotopyIterations=100  PhasorMode=off  PhasorModeNumHarmonics=1  DoDC=off  ResidualTolerance=1e-09  UseLocalSolver=off  LocalSolverChoice=NE_BACKWARD_EULER_ADVANCER  LocalSolverSampleTime=0.001  DoFixedCost=off  MaxNonlinIter=3  MaxModeIter=2  LinearAlgebra=Sparse  EquationFormulation=NE_TIME_EF  DelaysMemoryBudget=1024  AutomaticFiltering=on  FilteringTimeConstant=0.001  PartitionStorageMethod=AS_NEEDED  PartitionMemoryBudget=1024  PartitionMethod=FAST
  Velocity (deg/s) : Scope  Commented=on
  World Frame : sm_lib/Frames and Transforms/World Frame
  wires:
  Gain/1 -> Velocity (deg/s)/1
  THETA/1 -> Demux/1
  Demux/3 -> Simulink-PS Converter2/1
  PS-Simulink Converter/1 -> Gain/1
  Demux/2 -> Simulink-PS Converter1/1
  Demux/1 -> Simulink-PS Converter/1
  connections:
  Mechanism Configuration/RConn1 -- Solver Configuration/RConn1 -- World Frame/RConn1 -- Gimbal Joint/LConn1
  Gimbal Joint/LConn3 -- Simulink-PS Converter1/RConn1
  Gimbal Joint/LConn2 -- Simulink-PS Converter/RConn1
  CubeSat/RConn1 -- Gimbal Joint/RConn1
  Gimbal Joint/LConn4 -- Simulink-PS Converter2/RConn1

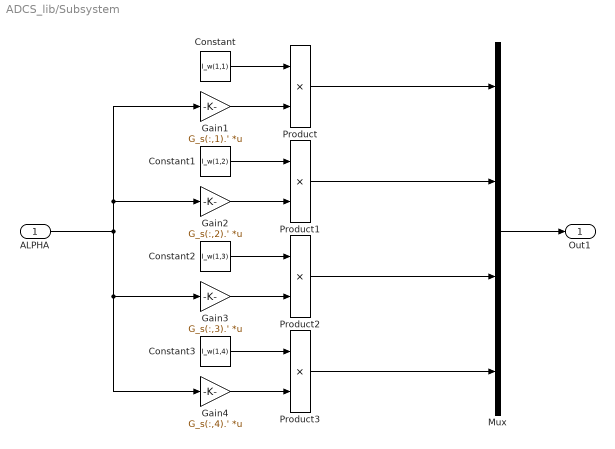
== system ADCS_lib/Subsystem ==
  ALPHA : Inport
  Constant : Constant  Value=I_w(1,1)
  Constant1 : Constant  Value=I_w(1,2)
  Constant2 : Constant  Value=I_w(1,3)
  Constant3 : Constant  Value=I_w(1,4)
  Gain1 : Gain  Gain=G_s(:,1).'  Multiplication=Matrix(K*u)
  Gain2 : Gain  Gain=G_s(:,2).'  Multiplication=Matrix(K*u)
  Gain3 : Gain  Gain=G_s(:,3).'  Multiplication=Matrix(K*u)
  Gain4 : Gain  Gain=G_s(:,4).'  Multiplication=Matrix(K*u)
  Mux : Mux
  Product{,1..3} (4 alike) : Product
  Out1 : Outport
  wires:
  ALPHA/1 -> Gain1/1, Gain2/1, Gain4/1, Gain3/1
  Gain1/1 -> Product/2
  Constant/1 -> Product/1
  Gain2/1 -> Product1/2
  Constant1/1 -> Product1/1
  Constant2/1 -> Product2/1
  Gain3/1 -> Product2/2
  Gain4/1 -> Product3/2
  Constant3/1 -> Product3/1
  Product/1 -> Mux/1
  Product1/1 -> Mux/2
  Product2/1 -> Mux/3
  Product3/1 -> Mux/4
  Mux/1 -> Out1/1
